simulink model "MC_R2_SFC_RELOJ_sin_antisway"  (R2025b)
settings: Solver=ode23t  StartTime=0.0  StopTime=600  MaxStep=T_s  RelTol=1e-4
InitFcn:
  | addpath(fileparts(get_param(bdroot,'FileName')),'-begin');
  | run(fullfile(fileparts(get_param(bdroot,'FileName')),'definir_buses_variadores.m'));
  | run(fullfile(fileparts(get_param(bdroot,'FileName')),'parametros_ganancias_cascada_29072026.m'));
  | run(fullfile(fileparts(get_param(bdroot,'FileName')),'configurar_modelo_final_hmi.m'));
  | run(fullfile(fileparts(get_param(bdroot,'FileName')),'configurar_parametros_variadores.m'));
  | Pvis.Ts_viz=0.04;Pvis.hmi.testDriver=@operador_medio_ciclo;
StopFcn:
  | cerrar_video_ensayo;
values from neighbouring files (symbols this model uses):
  MC_FF = struct('Ts',T_s,'gravity',g,'r_td',r_td,'i_t',i_t,'M_EQt',M_EQt,   'b_EQt',b_EQt,'Kx',K_x_cas,'Kp',K_pv_cas,'Ki',K_iv_cas,   'vmax',v_tmax,'amax',dv_tmax,'Imax',dv_tmax/K_iv_cas,   'r_hd',r_hd,'i_h',i_h,'M_EQh',M_EQh,'b_EQh',b_EQh,   'Khp',K_hp,'Khi',K_hi,'Khd',K_hd,'length0',l_hi,'swayOnTime',T_SW_on,   'swayFFRate',0.25,'observerWn',40.0,'observerZeta',1.0)    [configurar_parametros_variadores.m]
undefined symbols (not defined in the file or in its folder): b_cx, b_cy, b_hb, b_hEb, b_heq, b_t, b_tb, b_teq, b_tw, b_wu, g, H_c, HMI, i_h, i_t, J_heq, J_teq, K_cy, K_tw, k_wu, L_h0, l_hi, M_c_profile, M_s, M_t, nLevels0, omega_hmRATED, r_hd, r_td, slotBlock, T_hbMax, T_hEbMax, T_hmMax, T_s, T_s1, T_tbMax, T_tmMax, tau_hm, tau_tm, traj_duration, traj_x_start, traj_x_target, v_hmaxLoaded, v_hmaxUnloaded, x_tmax, x_tmin, Y_c0, Y_t0, Zbase
libraries: simulink x1, aerolibanimutils x1
(part 1 of 3)
Description:
  | Copia del modelo final con visualizacion y HMI integrada. Destino solo X, perfil LiDAR interno, offset de dos contenedores. Interfaz pasiva; retencion de barrido en supervisor. Correccion de ciclo: lazo de posicion de izaje, geometria real de slots, espera de alineacion/estabilidad y masa enclavada al PICK. Correccion de ciclo: lazo de posicion de izaje, geometria real de slots, espera de alineacion/estabilidad y masa enclavada al PICK. Correccion de ciclo: lazo de posicion de izaje, geometria real de slots, espera de alineacion/estabilidad y masa enclavada al PICK. Correccion de ciclo: lazo de posicion de izaje, geometria real de slots, espera de alineacion/estabilidad y masa enclavada al PICK. Correccion de ciclo: lazo de posicion de izaje, geometria real de slots, espera de alineacion/estabilidad y masa enclavada al PICK. Correccion de ciclo: lazo de posicion de izaje, geometria real de slots, espera de alineacion/estabilidad y masa enclavada al PICK. Correccion de ciclo: lazo de posicion de izaje, geometria real de slots, espera de alineacion/estabilidad y masa enclavada al PICK. Correccion de ciclo: lazo de posicion de izaje, geometria real de slots, espera de alineacion/estabilidad y masa enclavada al PICK. Correccion de ciclo: lazo de posicion de izaje, geometria real de slots, espera de alineacion/estabilidad y masa enclavada al PICK. Correccion de ciclo: lazo de posicion de izaje, geometria real de slots, espera de alineacion/estabilidad y masa enclavada al PICK. Correccion de ciclo: lazo de posicion de izaje, geometria real de slots, espera de alineacion/estabilidad y masa enclavada al PICK. Correccion de ciclo: lazo de posicion de izaje, geometria real de slots, espera de alineacion/estabilidad y masa enclavada al PICK.
  | Traslado productivo: 4 m/s y antisway inhibido durante transito con despeje confirmado.
  | Traslado productivo: 2.5 m/s y antisway inhibido durante crucero con despeje confirmado.
  | Traslado productivo: 2.5 m/s y antisway inhibido durante crucero con despeje confirmado.
settings Model: SimulationMode=accelerator  PacingRate=2  Creator=matie  LastModifiedBy=meesc
settings SolverCC: ZeroCrossAlgorithm=Adaptive  AlgebraicLoopSolver=TrustRegion
settings DataIOCC: SaveOutput=off  SaveTime=off
settings OptimizationCC: SimCompilerOptimization=on
settings DebuggingCC: IgnoredZcDiagnostic=none  UnconnectedInputMsg=warning  UnconnectedOutputMsg=warning  UnconnectedLineMsg=warning  BusObjectLabelMismatch=error
settings ModelReferenceCC: EnableRefExpFcnMdlSchedulingChecks=on
settings RTWCC: GPUComputeCapability=3.5
settings ConfigComp: PLC_OutputDir=C:\Temp\PLC_Code  PLC_TargetIDE=codesys23  PLC_MultiTBSigbuilderTimeRange=off  PLC_FoldFBCallOutputVar=off  PLC_RemoveUnusedSSMethodCallArguments=off  PLC_UseCallOutputArgSyntax=off  PLC_EnableUnsignedAndDoubleTypes=off  PLC_EnableUDTSplitting=off  PLC_MaxFieldsInUDT=500.0  PLC_InlineEnumCastFunction=off  PLC_RTWMaxIdLength=31.0  PLC_RollThreshold=5.0  PLC_ActiveTab=0.0  PLC_EnableStringLiteralTB=on  PLC_Enable64bitIntSupport=off

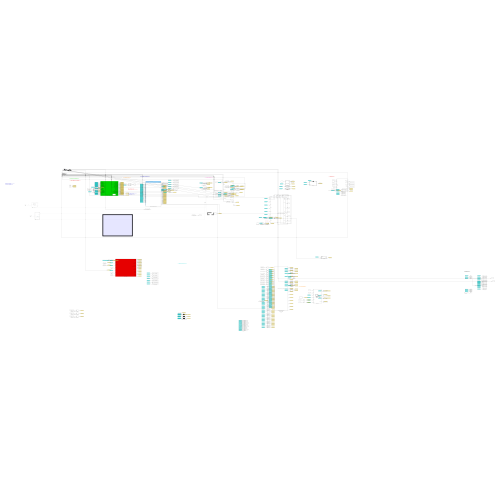
[thumbnail: Simulink's stored preview of the top-level diagram]
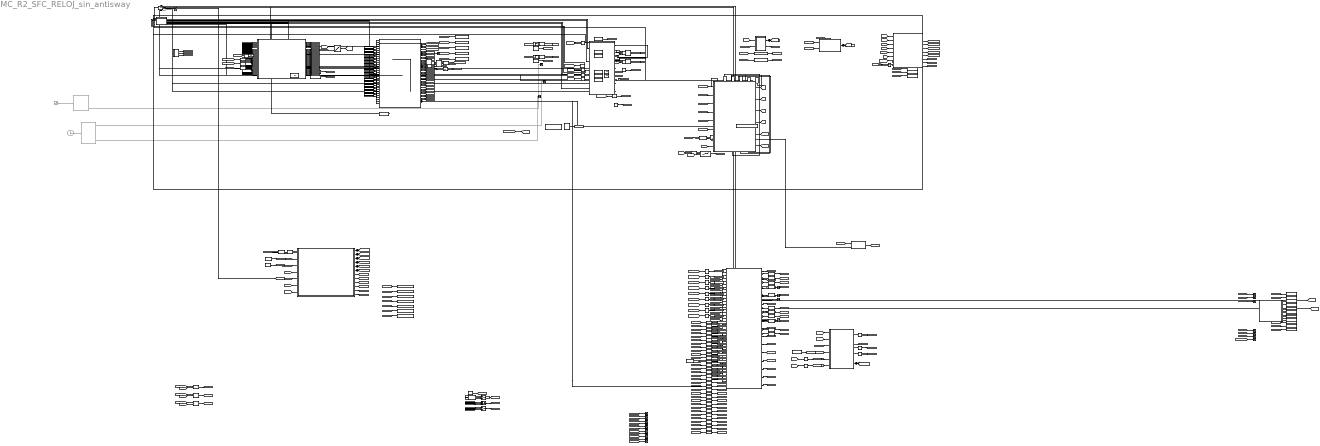
== system MC_R2_SFC_RELOJ_sin_antisway ==
  note: ESTIMADORES - OBSERVADORES
  note: INTEGRACION DEL SUPERVISOR
      | - Reemplaza exclusivamente Generador de trayectorias
      | - Conserva bloques comentados/no utilizados
      | - Ts supervisor: 20 ms; reguladores: 10 ms
  note: NIVEL 0 - SEGURIDAD (Ts = 20 ms)
      | E-stop/watchdog: emergencia total
      | Limite ultimo/sobrevelocidad: aislamiento selectivo por eje
  note: NIVEL 1 CORREGIDO - 2026-08-20
      | - Arranque automatico y planificador de obstaculos
      | - Transferencias bumpless
      | - Apertura de twistlocks y frenado seguro
  note: === INTERFAZ DE ENTRADAS ===
  note: === AUTOMATA SUPERVISOR ===
  note: === CONTROLADORES ===
  note: === PLANTA Y PERFIL ===
  note: === SENSORES ===
  note: === VISUALIZACION + HMI ===
  note: === AUTOMATA DE SEGURIDAD ===
  note: === TOMA / ENTREGA ===
  note: === MONITOREO ===
  1-D Lookup Table : Lookup_n-D  NumberOfTableDimensions=1  BreakpointsForDimension1=-30 + (0:32)*2.44  TableSource=Input port  Table=tanh([-5:5])  InterpMethod=Flat  InternalRulePriority=Speed  RndMeth=Simplest
      settings: InputPortMap=u0,p221
  Actualizar_Yc : Subsystem
  Altura cambio a automatico : Constant  Value=HMI.manualToAutoHeight
  Automata Supervisor : Subsystem
  Clock : Clock  Commented=on
  Consigna Izaje : MATLAB Function  Commented=on  TreatAsAtomicUnit=on
  Constant : Constant  Value=0
  Constant1 : Constant
  Constant2 : Constant  Value=l_hi
  Constant4 : Constant  Value=slotBlock
  Constant5 : Constant  Value=0
  Distancia aproximacion manual : Constant  Value=HMI.finalApproachDistance
  Estados MC carro : BusSelector  OutputSignals=x,omegaDrum,velocity,observerAngle
  Estados MC izaje : BusSelector  OutputSignals=length,lengthRate,omegaDrum,observerAngle
  HMI_COLISION_NO_DISPONIBLE : Constant  Value=NaN
  HMI_ESTADO_{10..41} (32 alike) : ZeroOrderHold  SampleTime=Pvis.Ts_viz
  HMI_MANDO_01 : DataTypeConversion  OutDataTypeStr=boolean  SaturateOnIntegerOverflow=off  RndMeth=Floor
  HMI_MANDO_02 : DataTypeConversion  OutDataTypeStr=boolean  SaturateOnIntegerOverflow=off  RndMeth=Floor
  HMI_MANDO_03 : DataTypeConversion  OutDataTypeStr=boolean  SaturateOnIntegerOverflow=off  RndMeth=Floor
  HMI_MANDO_04 : DataTypeConversion  OutDataTypeStr=boolean  SaturateOnIntegerOverflow=off  RndMeth=Floor
  HMI_MANDO_06 : DataTypeConversion  OutDataTypeStr=double  SaturateOnIntegerOverflow=off  RndMeth=Floor
  HMI_MANDO_09 : DataTypeConversion  OutDataTypeStr=boolean  SaturateOnIntegerOverflow=off  RndMeth=Floor
  HMI_MANDO_10 : DataTypeConversion  OutDataTypeStr=boolean  SaturateOnIntegerOverflow=off  RndMeth=Floor
  HMI_MANDO_11 : DataTypeConversion  OutDataTypeStr=boolean  SaturateOnIntegerOverflow=off  RndMeth=Floor
  HMI_MANDO_12 : DataTypeConversion  OutDataTypeStr=double  SaturateOnIntegerOverflow=off  RndMeth=Floor
  HMI_MANDO_14 : DataTypeConversion  OutDataTypeStr=double  SaturateOnIntegerOverflow=off  RndMeth=Floor
  HMI_MANDO_15 : DataTypeConversion  OutDataTypeStr=double  SaturateOnIntegerOverflow=off  RndMeth=Floor
  HMI_RESERVA_05 : Terminator
  HMI_RESERVA_07 : Terminator
  HMI_RESERVA_08 : Terminator
  HMI_RESERVA_13 : Terminator
  HMI_SELECT_JOY_H : Switch  Criteria=u2 > Threshold  Threshold=0.5  SaturateOnIntegerOverflow=off  InputSameDT=off
  HMI_SELECT_JOY_T : Switch  Criteria=u2 > Threshold  Threshold=0.5  SaturateOnIntegerOverflow=off  InputSameDT=off
  HMI_SELECT_TWIST_BUTTON : Switch  Criteria=u2 > Threshold  Threshold=0.5  SaturateOnIntegerOverflow=off  InputSameDT=off
  HMI_USE_JOYSTICK : Constant  Value=double(HMI.useJoystick)
  HMI_ZERO_INPUT : Constant  Value=0.0
  Habilitacion par izaje : Product  Inputs=**
  Habilitacion par trolley : Product  Inputs=**
  Histeresis_F_hw : MATLAB Function  TreatAsAtomicUnit=on
  Histeresis_contacto : MATLAB Function  TreatAsAtomicUnit=on
  Interfaz MC : Subsystem
  Interfaz de entradas del supervisor : Subsystem  Description=Interfaz pasiva: 33 conexiones directas Inport-Outport. Todo calculo y enclavamiento pertenece al automata supervisor.
  LIDAR_OFFSET_X : Bias  Bias=HMI.lidarOffsetX  SaturateOnIntegerOverflow=off
  LIDAR_PROFILE_LOOKUP : Lookup_n-D  NumberOfTableDimensions=1  BreakpointsForDimension1=-30 + (0:32)*2.44  TableSource=Input port  Table=tanh([-5:5])  InterpMethod=Flat  InternalRulePriority=Speed  RndMeth=Simplest
      settings: InputPortMap=u0,p221
  LOG_mon_aHoistMeasured : ToWorkspace  VariableName=mon_aHoistMeasured  SaveFormat=Timeseries  SampleTime=-1
  LOG_mon_aTrolleyMeasured : ToWorkspace  VariableName=mon_aTrolleyMeasured  SaveFormat=Timeseries  SampleTime=-1
  LOG_mon_automaticTargetY : ToWorkspace  VariableName=mon_automaticTargetY  SaveFormat=Timeseries  SampleTime=-1
  LOG_mon_ayRef : ToWorkspace  VariableName=mon_ayRef  SaveFormat=Timeseries  SampleTime=-1
  LOG_mon_contact4 : ToWorkspace  VariableName=mon_contact4  SaveFormat=Timeseries  SampleTime=-1
  LOG_mon_lidarX : ToWorkspace  VariableName=mon_lidarX  SaveFormat=Timeseries  SampleTime=-1
  LOG_mon_lidarY : ToWorkspace  VariableName=mon_lidarY  SaveFormat=Timeseries  SampleTime=-1
  LOG_mon_profileMaxY : ToWorkspace  VariableName=mon_profileMaxY  SaveFormat=Timeseries  SampleTime=-1
  LOG_mon_profileScanComplete : ToWorkspace  VariableName=mon_profileScanComplete  SaveFormat=Timeseries  SampleTime=-1
  LOG_mon_profileValid : ToWorkspace  VariableName=mon_profileValid  SaveFormat=Timeseries  SampleTime=-1
  LOG_mon_scanActive : ToWorkspace  VariableName=mon_scanActive  SaveFormat=Timeseries  SampleTime=-1
  LOG_mon_scannedObstacleProfile : ToWorkspace  VariableName=mon_scannedObstacleProfile  SaveFormat=Timeseries  SampleTime=-1
  LOG_mon_swayEnable : ToWorkspace  VariableName=mon_swayEnable  SaveFormat=Timeseries  SampleTime=-1
  LOG_mon_torqueProvenHoist : ToWorkspace  VariableName=mon_torqueProvenHoist  SaveFormat=Timeseries  SampleTime=-1
  LOG_mon_torqueProvenTrolley : ToWorkspace  VariableName=mon_torqueProvenTrolley  SaveFormat=Timeseries  SampleTime=-1
  LOG_mon_trackingFault : ToWorkspace  VariableName=mon_trackingFault  SaveFormat=Timeseries  SampleTime=-1
  LOG_mon_twistlockCloseCmd : ToWorkspace  VariableName=mon_twistlockCloseCmd  SaveFormat=Timeseries  SampleTime=-1
  LOG_mon_twistlocksClosed : ToWorkspace  VariableName=mon_twistlocksClosed  SaveFormat=Timeseries  SampleTime=-1
  LOG_mon_vyRef : ToWorkspace  VariableName=mon_vyRef  SaveFormat=Timeseries  SampleTime=-1
  LOG_mon_yRef : ToWorkspace  VariableName=mon_yRef  SaveFormat=Timeseries  SampleTime=-1
  LOG_n0_brakeHoistOpen : ToWorkspace  VariableName=n0_brakeHoistOpen  SaveFormat=Timeseries  SampleTime=-1
  LOG_n0_brakeTrolleyOpen : ToWorkspace  VariableName=n0_brakeTrolleyOpen  SaveFormat=Timeseries  SampleTime=-1
  LOG_n0_emergency : ToWorkspace  VariableName=n0_emergency  SaveFormat=Timeseries  SampleTime=-1
  LOG_n0_emergencyBrakeHoistOpen : ToWorkspace  VariableName=n0_emergencyBrakeHoistOpen  SaveFormat=Timeseries  SampleTime=-1
  LOG_n0_permitGlobal : ToWorkspace  VariableName=n0_permitGlobal  SaveFormat=Timeseries  SampleTime=-1
  LOG_n0_permitHoist : ToWorkspace  VariableName=n0_permitHoist  SaveFormat=Timeseries  SampleTime=-1
  LOG_n0_permitTrolley : ToWorkspace  VariableName=n0_permitTrolley  SaveFormat=Timeseries  SampleTime=-1
  LOG_sup_alarmCode : ToWorkspace  VariableName=sup_alarmCode  SaveFormat=Timeseries  SampleTime=-1
  LOG_sup_faultCode : ToWorkspace  VariableName=sup_faultCode  SaveFormat=Timeseries  SampleTime=-1
  LOG_sup_loadedState : ToWorkspace  VariableName=sup_loadedState  SaveFormat=Timeseries  SampleTime=-1
  LOG_sup_modeCode : ToWorkspace  VariableName=sup_modeCode  SaveFormat=Timeseries  SampleTime=-1
  LOG_sup_overloadDetected : ToWorkspace  VariableName=sup_overloadDetected  SaveFormat=Timeseries  SampleTime=-1
  MASS_latch_pick : MATLAB Function  TreatAsAtomicUnit=on
  MASS_loaded_gate : Product  Inputs=**
  MASS_profile_lookup : Lookup_n-D  NumberOfTableDimensions=1  BreakpointsForDimension1=1:33  Table=M_c_profile  InterpMethod=Flat  ExtrapMethod=Clip  InternalRulePriority=Speed  RndMeth=Simplest
  MASS_slot_double : DataTypeConversion  OutDataTypeStr=double  SaturateOnIntegerOverflow=off  RndMeth=Floor
  MONITOR_REQUISITOS : Subsystem
  Memoria recorte torque AW : UnitDelay  SampleTime=T_s  HasFrameUpgradeWarning=on
  Memory : Memory  InheritSampleTime=on
  Memory1 : Memory  InheritSampleTime=on
  Memory2 : Memory  InheritSampleTime=on
  Monitor bus diagnosticos 6 : Terminator
  Monitor bus diagnosticos 7 : Terminator
  Monitor estado carro {1..4} (4 alike) : Terminator
  Monitor estado izaje {1..4} (4 alike) : Terminator
  Motion Controller : Subsystem
  N0_CMD_ESTOP : Constant  Value=false  OutDataTypeStr=boolean
  N0_CMD_RESET : Constant  Value=false  OutDataTypeStr=boolean
  N0_GATE_BRK_H : Logic  AllPortsSameDT=off  OutDataTypeStr=boolean
  N0_GATE_BRK_HE : Logic  AllPortsSameDT=off  OutDataTypeStr=boolean
  N0_GATE_BRK_T : Logic  AllPortsSameDT=off  OutDataTypeStr=boolean
  N0_WATCHDOG_DELAY : UnitDelay  SampleTime=0.02  HasFrameUpgradeWarning=on
  N0_WATCHDOG_DOUBLE : DataTypeConversion  OutDataTypeStr=boolean  SaturateOnIntegerOverflow=off  RndMeth=Floor
  Nivel 0 - Seguridad : Subsystem
  PICK / PLACE : Stateflow chart  TreatAsAtomicUnit=on
      settings: PortSchema="{\"entries\":[{\"content\":{\"sides\":[{\"content\":{\"connectorIds\":[\"In1\",\"In4\",\"In2\",\"In3\",\"In5\",\"In6\"]},\"type\":\"ConnectorPlacement.EquallySpacedRectSide\",\"uuid\":\"a5c16d2a-5865-4365-aaee-c28e35544d9c\"},{\"content\":{\"connectorIds\":[\"Out1\",\"Out2\",\"Out3\",\"Out4\"],\"side\":\"RIGHT\"},\"type\":\"ConnectorPlacement.EquallySpacedRectSide\",\"uuid\":\"08faef91-0dc9-4101-b812-f759fd3bf652\"},{\"content\":{\"side\":\"TOP\"},\"type\":\"ConnectorPlacement.EquallySpacedRectSide\",\"uuid\":\"3d592ef8-c17c-453f-9fe4-450a9042f638\"}]},\"type\":\"ConnectorPlacement.EquallySpacedConnector\",\"uuid\":\"5bde2fb2-ef6e-4078-a945-4a946a0492f9\"}],\"packageUris\":[\"http://schema.mathworks.com/mf0/Connector/R2020b\"],\"version\":\"1.0\"}"
  Planta : Subsystem
      settings: PortSchema="{\"entries\":[{\"content\":{\"sides\":[{\"content\":{\"connectorIds\":[\"In1\",\"In2\",\"In3\",\"In4\",\"In5\",\"In6\",\"In7\",\"In8\"]},\"type\":\"ConnectorPlacement.EquallySpacedRectSide\",\"uuid\":\"5d76959f-b6a9-444d-8994-ab0bade83e0d\"},{\"content\":{\"connectorIds\":[\"Out1\",\"Out2\",\"Out3\",\"Out4\",\"Out5\",\"Out6\"],\"side\":\"RIGHT\"},\"type\":\"ConnectorPlacement.EquallySpacedRectSide\",\"uuid\":\"6304bef6-506d-485c-ab14-4271018549da\"},{\"content\":{\"connectorIds\":[\"Out7\",\"Out8\",\"Out9\",\"Out10\",\"Out11\",\"Out12\"],\"side\":\"TOP\"},\"type\":\"ConnectorPlacement.EquallySpacedRectSide\",\"uuid\":\"df87386f-05e1-445d-949d-2fc2ff55887c\"},{\"content\":{\"side\":\"BOTTOM\"},\"type\":\"ConnectorPlacement.EquallySpacedRectSide\",\"uuid\":\"6e66bc8d-e30f-453c-8c56-304efc1d1a44\"}]},\"type\":\"ConnectorPlacement.EquallySpacedConnector\",\"uuid\":\"ae511e70-0859-4f7f-ad0a-8f37dd26c1e0\"}],\"packageUris\":[\"http://schema.mathworks.com/mf0/Connector/R2020b\"],\"version\":\"1.0\"}"
  Push Button : PushButtonBlock  ButtonType=Latch  IconOnColor=[0.0, 0.39215686274509803, 0.0]  IconOffColor=[0.0, 1.0, 0.0]  OffValue=0.000000
  Registrar_envolvente_seguridad : ToWorkspace  VariableName=mon_safetyEnvelopeProfile  SaveFormat=Timeseries  SampleTime=-1
  SENSORES : Subsystem
  SUP_AUTO_TARGET_X_RAW : Constant  Value=HMI.shipTargetX  OutDataTypeStr=double
  SUP_CMD_AUTO_START_RAW : DataTypeConversion  OutDataTypeStr=boolean  SaturateOnIntegerOverflow=off  RndMeth=Floor
  SUP_CMD_AUTO_START_RAW_STEP : Step  Time=0.5  SampleTime=0
  SUP_CMD_RESET_RAW : Constant  Value=false  OutDataTypeStr=boolean
  SUP_CMD_START_RAW : DataTypeConversion  OutDataTypeStr=boolean  SaturateOnIntegerOverflow=off  RndMeth=Floor
  SUP_CMD_START_RAW_STEP : Step  Time=0.1  SampleTime=0
  SUP_CMD_STOP_RAW : Constant  Value=false  OutDataTypeStr=boolean
  SUP_CONFIG_VALID_RAW : Constant  Value=HMI.configValid  OutDataTypeStr=boolean
  SUP_CONTACT_BOOL : DataTypeConversion  OutDataTypeStr=boolean  SaturateOnIntegerOverflow=off  RndMeth=Floor
  SUP_FB_BOOL_7 : DataTypeConversion  OutDataTypeStr=boolean  SaturateOnIntegerOverflow=off  RndMeth=Floor
  SUP_FB_BOOL_8 : DataTypeConversion  OutDataTypeStr=boolean  SaturateOnIntegerOverflow=off  RndMeth=Floor
  SUP_MODE_AUTO_REQ_RAW : Constant  Value=HMI.modeAutoReq  OutDataTypeStr=boolean
  SUP_NOT_OPEN : Logic  Operator=NOT  AllPortsSameDT=off  OutDataTypeStr=boolean
  SUP_SCAN_PROFILE_REQ_RAW : Constant  Value=HMI.scanProfileReq  OutDataTypeStr=boolean
  SUP_SCAN_SPEED_RAW : Constant  Value=HMI.scanSpeed  OutDataTypeStr=double
  SUP_SWAY_SELECT_RAW : Constant  Value=HMI.swayControlSelect  OutDataTypeStr=boolean
  SUP_TLK_DOUBLE : DataTypeConversion  OutDataTypeStr=double  SaturateOnIntegerOverflow=off  RndMeth=Floor
  SUP_TLK_MEMORIA : UnitDelay  SampleTime=0.02  HasFrameUpgradeWarning=on
  SUP_TLK_SET_OR : Logic  Operator=OR  AllPortsSameDT=off  OutDataTypeStr=boolean
  SUP_TORQUE_HOIST_Z1 : UnitDelay  SampleTime=T_s1  HasFrameUpgradeWarning=on
  SUP_TORQUE_TROLLEY_Z1 : UnitDelay  SampleTime=T_s1  HasFrameUpgradeWarning=on
  SUP_TWISTLOCK_CMD : Logic  AllPortsSameDT=off  OutDataTypeStr=boolean
  SUP_TWISTLOCK_FB_DELAY : UnitDelay  SampleTime=0.02  HasFrameUpgradeWarning=on
  SW ultima muestra N1 : UnitDelay  SampleTime=T_s1  HasFrameUpgradeWarning=on
  Step : Step  Commented=on  Time=4  SampleTime=0
  Subsystem1 : Subsystem
  TERM_Constant : Terminator
  TERM_Constant1 : Terminator
  TERM_Constant5 : Terminator
  TERM_HMI_HMI_SELECT_JOY_H : Terminator
  TERM_HMI_HMI_SELECT_JOY_T : Terminator
  TERM_HMI_HMI_SELECT_TWIST_BUTTON : Terminator
  TERM_HMI_N0_CMD_ESTOP : Terminator
  TERM_HMI_N0_CMD_RESET : Terminator
  TERM_HMI_SUP_AUTO_TARGET_X_RAW : Terminator
  TERM_HMI_SUP_CMD_AUTO_START_RAW : Terminator
  TERM_HMI_SUP_CMD_RESET_RAW : Terminator
  TERM_HMI_SUP_CMD_START_RAW : Terminator
  TERM_HMI_SUP_CMD_STOP_RAW : Terminator
  TERM_HMI_SUP_MODE_AUTO_REQ_RAW : Terminator
  TERM_HMI_SUP_SCAN_PROFILE_REQ_RAW : Terminator
  TERM_SENSOR_08 : Terminator
  TERM_SENSOR_09 : Terminator
  TERM_SENSOR_10 : Terminator
  TERM_SUP_FB_6 : Terminator
  Terminator{2..5} (4 alike) : Terminator
  Transferencia antisway no transmitida : Terminator
  Transferencia no implementada PLC anterior : Constant  Value=0
  Trayectoria : Stateflow chart  Commented=on  TreatAsAtomicUnit=on  SystemSampleTime=1e-2
      settings: PortSchema="{\"entries\":[{\"content\":{\"sides\":[{\"content\":{\"connectorIds\":[\"In1\"]},\"type\":\"ConnectorPlacement.EquallySpacedRectSide\",\"uuid\":\"6f391abb-7914-46b1-bf75-00dd597d8745\"},{\"content\":{\"connectorIds\":[\"Out2\",\"Out1\",\"Out3\",\"Out4\"],\"side\":\"RIGHT\"},\"type\":\"ConnectorPlacement.EquallySpacedRectSide\",\"uuid\":\"48dcce50-4b02-4ca8-9f00-9379aa6a7819\"},{\"content\":{\"side\":\"TOP\"},\"type\":\"ConnectorPlacement.EquallySpacedRectSide\",\"uuid\":\"d392ffd4-6ceb-4d84-99b2-b6bd8ae66add\"}]},\"type\":\"ConnectorPlacement.EquallySpacedConnector\",\"uuid\":\"17183b69-1a6f-4f40-a08d-c34759601e28\"}],\"packageUris\":[\"http://schema.mathworks.com/mf0/Connector/R2020b\"],\"version\":\"1.0\"}"
  Unit Delay : UnitDelay  SampleTime=-1  HasFrameUpgradeWarning=on
  Unit Delay1 : UnitDelay  SampleTime=-1  HasFrameUpgradeWarning=on
  VIS ZOH 01 : ZeroOrderHold  SampleTime=Pvis.Ts_viz
  VIS ZOH 02 : ZeroOrderHold  SampleTime=Pvis.Ts_viz
  VIS ZOH 03 : ZeroOrderHold  SampleTime=Pvis.Ts_viz
  VIS ZOH 04 : ZeroOrderHold  SampleTime=Pvis.Ts_viz
  VIS ZOH 05 : ZeroOrderHold  SampleTime=Pvis.Ts_viz
  VIS ZOH 06 : ZeroOrderHold  SampleTime=Pvis.Ts_viz
  VIS ZOH 07 : ZeroOrderHold  SampleTime=Pvis.Ts_viz
  VIS ZOH 08 : ZeroOrderHold  SampleTime=Pvis.Ts_viz
  VIS ZOH 09 : ZeroOrderHold  SampleTime=Pvis.Ts_viz
  VISUALIZACION 2D SISTEMA GRUA : M-S-Function  FunctionName=visualizacion_modelo_final_hmi_corregido
      settings: AttributesFormatString=Grua + HMI interactiva\n41 estados / 15 mandos\nTs = 40 ms
  Zero-Order Hold{,5..10} (7 alike) : ZeroOrderHold  SampleTime=T_s
  Zero-Order Hold11 : ZeroOrderHold  SampleTime=0.001
  Zero-Order Hold12 : ZeroOrderHold  SampleTime=0.001
  slot_x_l : MATLAB Function  TreatAsAtomicUnit=on
  tag scope: F_hw=global, N0_BRK_H=global, N0_BRK_HE=global, N0_BRK_T=global, N0_PERMIT_GLOBAL=global, N0_PERMIT_HOIST=global, N0_PERMIT_TROLLEY=global, Y_c=global, a_tgen=global, carga_tomada=global, k_slot=global, omega_l=global, theta_l=global, v_ly=global, v_tgen=global, x_t=global, x_tgen=global, y_l=global
  wires:
  Step/1 -> Trayectoria/1(iniciar)  "start"
  Trayectoria/4(j_act) -> Terminator5/1
  1-D Lookup Table/1 -> [yc_xl]
  Clock/1 -> Consigna Izaje/1(t)
  Consigna Izaje/1(lh_ref) -> Terminator2/1  "lh_ref"
  Consigna Izaje/4(done) -> Terminator4/1
  Actualizar_Yc/1(Y_c) -> [Y_c], [TOP_Actualizar_Yc_P1]
  Altura cambio a automatico/1 -> [TOP_Altura_cambio_a_automatico_P1]
  Constant/1 -> [TOP_Constant_P1]
  Constant1/1 -> [TOP_Constant1_P1]
  Constant4/1 -> [TOP_Constant4_P1]
  Constant5/1 -> [TOP_Constant5_P1]
  Distancia aproximacion manual/1 -> [TOP_Distancia_aproximacion_manual_P1]
  [theta_l_sens] -> Zero-Order Hold5/1
  [F_hw] -> Zero-Order Hold12/1
  [yc_xl] -> Planta/8(y_c0(x_l,t))  "yc_xl"
  [x_l] -> slot_x_l/1(x_l)
  [x_l] -> 1-D Lookup Table/1
  [x_tgen] -> Zero-Order Hold6/1
  [carga_tomada] -> Unit Delay/1
  [TLK] -> PICK / PLACE/1(TLK)
  [theta_l] -> SENSORES/4(theta_l)
  [x_t] -> SENSORES/6(x_t)
  [omega_hd] -> SENSORES/7(In7)
  [theta_tm] -> SENSORES/1(In1)
  [theta_hm] -> SENSORES/2(In2)
  [F_hw] -> SENSORES/3(In3)
  [v_tgen] -> Zero-Order Hold7/1
  [omega_l] -> SENSORES/5(omega_l)
  [carga_tomada] -> Unit Delay1/1
  [v_ly] -> PICK / PLACE/4(v_yl)
  [F_cy] -> Zero-Order Hold11/1
  [a_tgen] -> Zero-Order Hold8/1
  [F_hw_sens] -> Zero-Order Hold/1
  [TOP_Actualizar_Yc_P1] -> 1-D Lookup Table/2
  [TOP_Altura_cambio_a_automatico_P1] -> Interfaz de entradas del supervisor/26(IN_26_manualToAutoHeight)
  [TOP_Automata_Supervisor_P10] -> HMI_ESTADO_23/1
  [TOP_Automata_Supervisor_P10] -> LOG_sup_overloadDetected/1
  [TOP_Automata_Supervisor_P11] -> N0_WATCHDOG_DOUBLE/1
  [TOP_Automata_Supervisor_P15] -> LOG_mon_yRef/1
  [TOP_Automata_Supervisor_P15] -> Terminator3/1
  [TOP_Automata_Supervisor_P16] -> LOG_mon_vyRef/1
  [TOP_Automata_Supervisor_P17] -> LOG_mon_ayRef/1
  [TOP_Automata_Supervisor_P18] -> HMI_ESTADO_10/1
  [TOP_Automata_Supervisor_P18] -> LOG_sup_modeCode/1
  [TOP_Automata_Supervisor_P19] -> LOG_sup_alarmCode/1
  [TOP_Automata_Supervisor_P20] -> HMI_ESTADO_40/1
  [TOP_Automata_Supervisor_P20] -> LOG_sup_faultCode/1
  [TOP_Automata_Supervisor_P21] -> LOG_mon_aTrolleyMeasured/1
  [TOP_Automata_Supervisor_P22] -> LOG_mon_aHoistMeasured/1
  [TOP_Automata_Supervisor_P23] -> HMI_ESTADO_39/1
  [TOP_Automata_Supervisor_P23] -> LOG_mon_trackingFault/1
  [TOP_Automata_Supervisor_P24] -> LOG_mon_torqueProvenTrolley/1
  [TOP_Automata_Supervisor_P25] -> LOG_mon_torqueProvenHoist/1
  [TOP_Automata_Supervisor_P26] -> HMI_ESTADO_41/1
  [TOP_Automata_Supervisor_P26] -> LOG_mon_profileScanComplete/1
  [TOP_Automata_Supervisor_P27] -> HMI_ESTADO_37/1
  [TOP_Automata_Supervisor_P27] -> LOG_mon_profileValid/1
  [TOP_Automata_Supervisor_P28] -> HMI_ESTADO_38/1
  [TOP_Automata_Supervisor_P28] -> LOG_mon_scanActive/1
  [TOP_Automata_Supervisor_P29] -> LOG_mon_scannedObstacleProfile/1
  [TOP_Automata_Supervisor_P30] -> LOG_mon_profileMaxY/1
  [TOP_Automata_Supervisor_P31] -> HMI_ESTADO_36/1
  [TOP_Automata_Supervisor_P31] -> LOG_mon_automaticTargetY/1
  [TOP_Automata_Supervisor_P32] -> HMI_ESTADO_35/1
  [TOP_Automata_Supervisor_P33] -> HMI_ESTADO_12/1
  [TOP_Automata_Supervisor_P34] -> HMI_ESTADO_13/1
  [TOP_Automata_Supervisor_P35] -> HMI_ESTADO_26/1
  [TOP_Automata_Supervisor_P36] -> HMI_ESTADO_27/1
  [TOP_Automata_Supervisor_P37] -> HMI_ESTADO_20/1
  [TOP_Automata_Supervisor_P38] -> HMI_ESTADO_21/1
  [TOP_Automata_Supervisor_P6] -> LOG_mon_twistlockCloseCmd/1
  [TOP_Automata_Supervisor_P6] -> SUP_TLK_SET_OR/1
  [TOP_Automata_Supervisor_P7] -> SUP_NOT_OPEN/1
  [TOP_Automata_Supervisor_P8] -> HMI_ESTADO_14/1
  [TOP_Automata_Supervisor_P8] -> LOG_mon_swayEnable/1
  [TOP_Automata_Supervisor_P9] -> LOG_sup_loadedState/1
  [TOP_Constant1_P1] -> TERM_Constant1/1
  [TOP_Constant4_P1] -> slot_x_l/2(slotBlock)
  [TOP_Constant5_P1] -> TERM_Constant5/1
  [TOP_Constant_P1] -> TERM_Constant/1
  [TOP_Distancia_aproximacion_manual_P1] -> Interfaz de entradas del supervisor/27(IN_27_finalApproachDistance)
  [TOP_HMI_COLISION_NO_DISPONIBLE_P1] -> HMI_ESTADO_28/1
  [TOP_HMI_ESTADO_10_P1] -> VISUALIZACION 2D SISTEMA GRUA/10
  [TOP_HMI_ESTADO_11_P1] -> VISUALIZACION 2D SISTEMA GRUA/11
  [TOP_HMI_ESTADO_12_P1] -> VISUALIZACION 2D SISTEMA GRUA/12
  [TOP_HMI_ESTADO_13_P1] -> VISUALIZACION 2D SISTEMA GRUA/13
  [TOP_HMI_ESTADO_14_P1] -> VISUALIZACION 2D SISTEMA GRUA/14
  [TOP_HMI_ESTADO_15_P1] -> VISUALIZACION 2D SISTEMA GRUA/15
  [TOP_HMI_ESTADO_16_P1] -> VISUALIZACION 2D SISTEMA GRUA/16
  [TOP_HMI_ESTADO_17_P1] -> VISUALIZACION 2D SISTEMA GRUA/17
  [TOP_HMI_ESTADO_18_P1] -> VISUALIZACION 2D SISTEMA GRUA/18
  [TOP_HMI_ESTADO_19_P1] -> VISUALIZACION 2D SISTEMA GRUA/19
  [TOP_HMI_ESTADO_20_P1] -> VISUALIZACION 2D SISTEMA GRUA/20
  [TOP_HMI_ESTADO_21_P1] -> VISUALIZACION 2D SISTEMA GRUA/21
  [TOP_HMI_ESTADO_22_P1] -> VISUALIZACION 2D SISTEMA GRUA/22
  [TOP_HMI_ESTADO_23_P1] -> VISUALIZACION 2D SISTEMA GRUA/23
  [TOP_HMI_ESTADO_24_P1] -> VISUALIZACION 2D SISTEMA GRUA/24
  [TOP_HMI_ESTADO_25_P1] -> VISUALIZACION 2D SISTEMA GRUA/25
  [TOP_HMI_ESTADO_26_P1] -> VISUALIZACION 2D SISTEMA GRUA/26
  [TOP_HMI_ESTADO_27_P1] -> VISUALIZACION 2D SISTEMA GRUA/27
  [TOP_HMI_ESTADO_28_P1] -> VISUALIZACION 2D SISTEMA GRUA/28
  [TOP_HMI_ESTADO_29_P1] -> VISUALIZACION 2D SISTEMA GRUA/29
  [TOP_HMI_ESTADO_30_P1] -> VISUALIZACION 2D SISTEMA GRUA/30
  [TOP_HMI_ESTADO_31_P1] -> VISUALIZACION 2D SISTEMA GRUA/31
  [TOP_HMI_ESTADO_32_P1] -> VISUALIZACION 2D SISTEMA GRUA/32
  [TOP_HMI_ESTADO_33_P1] -> VISUALIZACION 2D SISTEMA GRUA/33
  [TOP_HMI_ESTADO_34_P1] -> VISUALIZACION 2D SISTEMA GRUA/34
  [TOP_HMI_ESTADO_35_P1] -> VISUALIZACION 2D SISTEMA GRUA/35
  [TOP_HMI_ESTADO_36_P1] -> VISUALIZACION 2D SISTEMA GRUA/36
  [TOP_HMI_ESTADO_37_P1] -> VISUALIZACION 2D SISTEMA GRUA/37
  [TOP_HMI_ESTADO_38_P1] -> VISUALIZACION 2D SISTEMA GRUA/38
  [TOP_HMI_ESTADO_39_P1] -> VISUALIZACION 2D SISTEMA GRUA/39
  [TOP_HMI_ESTADO_40_P1] -> VISUALIZACION 2D SISTEMA GRUA/40
  [TOP_HMI_ESTADO_41_P1] -> VISUALIZACION 2D SISTEMA GRUA/41
  [TOP_HMI_MANDO_01_P1] -> Interfaz de entradas del supervisor/1(IN_01_cmdStart)
  [TOP_HMI_MANDO_02_P1] -> Interfaz de entradas del supervisor/2(IN_02_cmdStop)
  [TOP_HMI_MANDO_03_P1] -> Nivel 0 - Seguridad/3(emergencyStop)
  [TOP_HMI_MANDO_04_P1] -> Interfaz de entradas del supervisor/30(IN_30_scanProfileReq)
  [TOP_HMI_MANDO_06_P1] -> Interfaz de entradas del supervisor/25(IN_25_autoTargetX)
  [TOP_HMI_MANDO_09_P1] -> Interfaz de entradas del supervisor/3(IN_03_modeAutoReq)
  [TOP_HMI_MANDO_10_P1] -> Interfaz de entradas del supervisor/4(IN_04_cmdAutoStart)
  [TOP_HMI_MANDO_11_P1] -> Interfaz de entradas del supervisor/5(IN_05_cmdReset)
  [TOP_HMI_MANDO_11_P1] -> Nivel 0 - Seguridad/2(resetSafety)
  [TOP_HMI_MANDO_12_P1] -> Interfaz de entradas del supervisor/8(IN_08_twistlockButton)
  [TOP_HMI_MANDO_14_P1] -> Interfaz de entradas del supervisor/16(IN_16_joyTrolley)
  [TOP_HMI_MANDO_15_P1] -> Interfaz de entradas del supervisor/17(IN_17_joyHoist)
  [TOP_HMI_SELECT_JOY_H_P1] -> TERM_HMI_HMI_SELECT_JOY_H/1
  [TOP_HMI_SELECT_JOY_T_P1] -> TERM_HMI_HMI_SELECT_JOY_T/1
  [TOP_HMI_SELECT_TWIST_BUTTON_P1] -> TERM_HMI_HMI_SELECT_TWIST_BUTTON/1
  [TOP_HMI_USE_JOYSTICK_P1] -> HMI_SELECT_JOY_H/2
  [TOP_HMI_USE_JOYSTICK_P1] -> HMI_SELECT_JOY_T/2
  [TOP_HMI_USE_JOYSTICK_P1] -> HMI_SELECT_TWIST_BUTTON/2
  [TOP_HMI_ZERO_INPUT_P1] -> HMI_SELECT_JOY_H/3
  [TOP_HMI_ZERO_INPUT_P1] -> HMI_SELECT_JOY_T/3
  [TOP_HMI_ZERO_INPUT_P1] -> HMI_SELECT_TWIST_BUTTON/3
  [TOP_Habilitacion_par_izaje_P1] -> Planta/1(T_hm*)
  [TOP_Habilitacion_par_trolley_P1] -> Planta/2(T_tm*)
  [TOP_Histeresis_F_hw_P1] -> PICK / PLACE/6(tension)
  [TOP_Histeresis_contacto_P1] -> PICK / PLACE/5(contacto)
  [TOP_Histeresis_contacto_P1] -> SUP_CONTACT_BOOL/1
  [TOP_Interfaz_de_entradas_del_supervisor_P9] -> LOG_mon_contact4/1
  [TOP_Interfaz_de_entradas_del_supervisor_P9] -> HMI_ESTADO_11/1
  [TOP_Interfaz_de_entradas_del_supervisor_P10] -> LOG_mon_twistlocksClosed/1
  [TOP_Interfaz_de_entradas_del_supervisor_P11] -> HMI_ESTADO_24/1
  [TOP_Interfaz_de_entradas_del_supervisor_P12] -> HMI_ESTADO_25/1
  [TOP_Interfaz_de_entradas_del_supervisor_P16] -> HMI_ESTADO_18/1
  [TOP_Interfaz_de_entradas_del_supervisor_P17] -> HMI_ESTADO_19/1
  [TOP_Interfaz_de_entradas_del_supervisor_P3] -> HMI_ESTADO_30/1
  [TOP_Interfaz_de_entradas_del_supervisor_P31] -> LOG_mon_lidarX/1
  [TOP_Interfaz_de_entradas_del_supervisor_P32] -> LOG_mon_lidarY/1
  [TOP_LIDAR_OFFSET_X_P1] -> Interfaz de entradas del supervisor/31(IN_31_lidarX)
  [TOP_LIDAR_OFFSET_X_P1] -> LIDAR_PROFILE_LOOKUP/1
  [TOP_LIDAR_PROFILE_LOOKUP_P1] -> Interfaz de entradas del supervisor/32(IN_32_lidarY)
  [TOP_MASS_latch_pick_P1] -> MASS_loaded_gate/1
  [TOP_MASS_loaded_gate_P1] -> Planta/7(M_c)
  [TOP_MASS_profile_lookup_P1] -> MASS_latch_pick/1(profileMass)
  [TOP_MASS_slot_double_P1] -> MASS_profile_lookup/1
  [TOP_Memory1_P1] -> Actualizar_Yc/1(tipo_evento)
  [TOP_Memory2_P1] -> Actualizar_Yc/2(slot_evento)
  [TOP_Memory_P1] -> Actualizar_Yc/Trigger
  [TOP_N0_CMD_ESTOP_P1] -> TERM_HMI_N0_CMD_ESTOP/1
  [TOP_N0_CMD_RESET_P1] -> TERM_HMI_N0_CMD_RESET/1
  [TOP_N0_GATE_BRK_HE_P1] -> Planta/4(BRK_hE)
  [TOP_N0_GATE_BRK_H_P1] -> Planta/5(BRK_h)
  [TOP_N0_GATE_BRK_T_P1] -> Planta/3(BRK_t)
  [TOP_N0_OMEGA_A_VT_P1] -> Nivel 0 - Seguridad/5(vTrolley)
  [TOP_N0_WATCHDOG_DELAY_P1] -> Nivel 0 - Seguridad/1(watchdogPulse)
  [TOP_N0_WATCHDOG_DOUBLE_P1] -> N0_WATCHDOG_DELAY/1
  [TOP_Nivel_0_Seguridad_P10] -> HMI_ESTADO_32/1
  [TOP_Nivel_0_Seguridad_P11] -> HMI_ESTADO_33/1
  [TOP_Nivel_0_Seguridad_P12] -> HMI_ESTADO_34/1
  [TOP_Nivel_0_Seguridad_P1] -> LOG_n0_permitGlobal/1
  [TOP_Nivel_0_Seguridad_P2] -> LOG_n0_permitTrolley/1
  [TOP_Nivel_0_Seguridad_P3] -> LOG_n0_permitHoist/1
  [TOP_Nivel_0_Seguridad_P4] -> HMI_ESTADO_15/1
  [TOP_Nivel_0_Seguridad_P4] -> LOG_n0_brakeTrolleyOpen/1
  [TOP_Nivel_0_Seguridad_P5] -> HMI_ESTADO_16/1
  [TOP_Nivel_0_Seguridad_P5] -> LOG_n0_brakeHoistOpen/1
  [TOP_Nivel_0_Seguridad_P6] -> HMI_ESTADO_17/1
  [TOP_Nivel_0_Seguridad_P6] -> LOG_n0_emergencyBrakeHoistOpen/1
  [TOP_Nivel_0_Seguridad_P7] -> HMI_ESTADO_22/1
  [TOP_Nivel_0_Seguridad_P7] -> LOG_n0_emergency/1
  [TOP_Nivel_0_Seguridad_P8] -> HMI_ESTADO_29/1
  [TOP_Nivel_0_Seguridad_P9] -> HMI_ESTADO_31/1
  [TOP_PICK_PLACE_P1] -> Memory/1
  [TOP_PICK_PLACE_P2] -> Memory1/1
  [TOP_PICK_PLACE_P3] -> Memory2/1
  [TOP_PICK_PLACE_P4] -> MASS_loaded_gate/2, MASS_latch_pick/2(loaded)
  [TOP_SENSORES_P10] -> TERM_SENSOR_10/1
  [TOP_SENSORES_P8] -> TERM_SENSOR_08/1
  [TOP_SENSORES_P9] -> TERM_SENSOR_09/1
  [TOP_SUP_AUTO_TARGET_X_RAW_P1] -> TERM_HMI_SUP_AUTO_TARGET_X_RAW/1
  [TOP_SUP_CMD_AUTO_START_RAW_P1] -> TERM_HMI_SUP_CMD_AUTO_START_RAW/1
  [TOP_SUP_CMD_AUTO_START_RAW_STEP_P1] -> SUP_CMD_AUTO_START_RAW/1
  [TOP_SUP_CMD_RESET_RAW_P1] -> TERM_HMI_SUP_CMD_RESET_RAW/1
  [TOP_SUP_CMD_START_RAW_P1] -> TERM_HMI_SUP_CMD_START_RAW/1
  [TOP_SUP_CMD_START_RAW_STEP_P1] -> SUP_CMD_START_RAW/1
  [TOP_SUP_CMD_STOP_RAW_P1] -> TERM_HMI_SUP_CMD_STOP_RAW/1
  [TOP_SUP_CONFIG_VALID_RAW_P1] -> Interfaz de entradas del supervisor/7(IN_07_configValid)
  [TOP_SUP_CONTACT_BOOL_P1] -> Interfaz de entradas del supervisor/9(IN_09_contact4)
  [TOP_SUP_FB_BOOL_7_P1] -> Interfaz de entradas del supervisor/11(IN_11_normalLimitXMin)
  [TOP_SUP_FB_BOOL_8_P1] -> Interfaz de entradas del supervisor/12(IN_12_normalLimitXMax)
  [TOP_SUP_MODE_AUTO_REQ_RAW_P1] -> TERM_HMI_SUP_MODE_AUTO_REQ_RAW/1
  [TOP_SUP_NOT_OPEN_P1] -> SUP_TWISTLOCK_CMD/2
  [TOP_SUP_SCAN_PROFILE_REQ_RAW_P1] -> TERM_HMI_SUP_SCAN_PROFILE_REQ_RAW/1
  [TOP_SUP_SCAN_SPEED_RAW_P1] -> Interfaz de entradas del supervisor/33(IN_33_scanSpeed)
  [TOP_SUP_SWAY_SELECT_RAW_P1] -> Interfaz de entradas del supervisor/6(IN_06_swayControlSelect)
  [TOP_SUP_TLK_MEMORIA_P1] -> SUP_TLK_SET_OR/2
  [TOP_SUP_TLK_MEMORIA_P1] -> SUP_TWISTLOCK_FB_DELAY/1
  [TOP_SUP_TLK_SET_OR_P1] -> SUP_TWISTLOCK_CMD/1
  [TOP_SUP_TORQUE_HOIST_Z1_P1] -> Interfaz de entradas del supervisor/24(IN_24_torqueHoistRaw)
  [TOP_SUP_TORQUE_TROLLEY_Z1_P1] -> Interfaz de entradas del supervisor/23(IN_23_torqueTrolleyRaw)
  [TOP_SUP_TWISTLOCK_CMD_P1] -> SUP_TLK_DOUBLE/1
  [TOP_SUP_TWISTLOCK_CMD_P1] -> SUP_TLK_MEMORIA/1
  [TOP_SUP_TWISTLOCK_FB_DELAY_P1] -> Interfaz de entradas del supervisor/10(IN_10_twistlocksClosedFb)
  [TOP_Subsystem1_P1] -> HMI_SELECT_TWIST_BUTTON/1
  [TOP_Subsystem1_P2] -> HMI_SELECT_JOY_H/1
  [TOP_Subsystem1_P3] -> HMI_SELECT_JOY_T/1
  [TOP_Subsystem_P1] -> SUP_TORQUE_HOIST_Z1/1
  [TOP_Subsystem_P1] -> Zero-Order Hold9/1
  [TOP_Subsystem_P2] -> SUP_TORQUE_TROLLEY_Z1/1
  [TOP_Subsystem_P2] -> Zero-Order Hold10/1
  [TOP_Unit_Delay1_P1] -> SENSORES/8(TLK)
  [TOP_Unit_Delay_P1] -> Planta/6(TLK)
  [TOP_VISUALIZACION_2D_SISTEMA_GRUA_P10] -> HMI_MANDO_10/1
  [TOP_VISUALIZACION_2D_SISTEMA_GRUA_P11] -> HMI_MANDO_11/1
  [TOP_VISUALIZACION_2D_SISTEMA_GRUA_P12] -> HMI_MANDO_12/1
  [TOP_VISUALIZACION_2D_SISTEMA_GRUA_P13] -> HMI_RESERVA_13/1
  [TOP_VISUALIZACION_2D_SISTEMA_GRUA_P14] -> HMI_MANDO_14/1
  [TOP_VISUALIZACION_2D_SISTEMA_GRUA_P15] -> HMI_MANDO_15/1
  [TOP_VISUALIZACION_2D_SISTEMA_GRUA_P1] -> HMI_MANDO_01/1
  [TOP_VISUALIZACION_2D_SISTEMA_GRUA_P2] -> HMI_MANDO_02/1
  [TOP_VISUALIZACION_2D_SISTEMA_GRUA_P3] -> HMI_MANDO_03/1
  [TOP_VISUALIZACION_2D_SISTEMA_GRUA_P4] -> HMI_MANDO_04/1
  [TOP_VISUALIZACION_2D_SISTEMA_GRUA_P5] -> HMI_RESERVA_05/1
  [TOP_VISUALIZACION_2D_SISTEMA_GRUA_P6] -> HMI_MANDO_06/1
  [TOP_VISUALIZACION_2D_SISTEMA_GRUA_P7] -> HMI_RESERVA_07/1
  [TOP_VISUALIZACION_2D_SISTEMA_GRUA_P8] -> HMI_RESERVA_08/1
  [TOP_VISUALIZACION_2D_SISTEMA_GRUA_P9] -> HMI_MANDO_09/1
  [TOP_VIS_ZOH_01_P1] -> VISUALIZACION 2D SISTEMA GRUA/1
  [TOP_VIS_ZOH_02_P1] -> VISUALIZACION 2D SISTEMA GRUA/2
  [TOP_VIS_ZOH_03_P1] -> VISUALIZACION 2D SISTEMA GRUA/3
  [TOP_VIS_ZOH_04_P1] -> VISUALIZACION 2D SISTEMA GRUA/4
  [TOP_VIS_ZOH_05_P1] -> VISUALIZACION 2D SISTEMA GRUA/5
  [TOP_VIS_ZOH_06_P1] -> VISUALIZACION 2D SISTEMA GRUA/6
  [TOP_VIS_ZOH_07_P1] -> VISUALIZACION 2D SISTEMA GRUA/7
  [TOP_VIS_ZOH_08_P1] -> VISUALIZACION 2D SISTEMA GRUA/8
  [TOP_VIS_ZOH_09_P1] -> VISUALIZACION 2D SISTEMA GRUA/9
  [TOP_Zero_Order_Hold10_P1] -> Habilitacion par trolley/1
  [TOP_Zero_Order_Hold11_P1] -> Histeresis_contacto/1(F_cy)
  [TOP_Zero_Order_Hold12_P1] -> Histeresis_F_hw/1(F_hw)
  [TOP_Zero_Order_Hold9_P1] -> Habilitacion par izaje/1
  [TOP_slot_x_l_P1] -> MASS_slot_double/1
  [TOP_slot_x_l_P1] -> PICK / PLACE/2(k_slot)
  [TOP_slot_x_l_P2] -> PICK / PLACE/3(slot_ok)
  HMI_COLISION_NO_DISPONIBLE/1 -> [TOP_HMI_COLISION_NO_DISPONIBLE_P1]
  HMI_ESTADO_10/1 -> [TOP_HMI_ESTADO_10_P1]
  HMI_ESTADO_11/1 -> [TOP_HMI_ESTADO_11_P1]
  HMI_ESTADO_12/1 -> [TOP_HMI_ESTADO_12_P1]
  HMI_ESTADO_13/1 -> [TOP_HMI_ESTADO_13_P1]
  HMI_ESTADO_14/1 -> [TOP_HMI_ESTADO_14_P1]
  HMI_ESTADO_15/1 -> [TOP_HMI_ESTADO_15_P1]
  HMI_ESTADO_16/1 -> [TOP_HMI_ESTADO_16_P1]
  HMI_ESTADO_17/1 -> [TOP_HMI_ESTADO_17_P1]
  HMI_ESTADO_18/1 -> [TOP_HMI_ESTADO_18_P1]
  HMI_ESTADO_19/1 -> [TOP_HMI_ESTADO_19_P1]
  HMI_ESTADO_20/1 -> [TOP_HMI_ESTADO_20_P1]
  HMI_ESTADO_21/1 -> [TOP_HMI_ESTADO_21_P1]
  HMI_ESTADO_22/1 -> [TOP_HMI_ESTADO_22_P1]
  HMI_ESTADO_23/1 -> [TOP_HMI_ESTADO_23_P1]
  HMI_ESTADO_24/1 -> [TOP_HMI_ESTADO_24_P1]
  HMI_ESTADO_25/1 -> [TOP_HMI_ESTADO_25_P1]
  HMI_ESTADO_26/1 -> [TOP_HMI_ESTADO_26_P1]
  HMI_ESTADO_27/1 -> [TOP_HMI_ESTADO_27_P1]
  HMI_ESTADO_28/1 -> [TOP_HMI_ESTADO_28_P1]
  HMI_ESTADO_29/1 -> [TOP_HMI_ESTADO_29_P1]
  HMI_ESTADO_30/1 -> [TOP_HMI_ESTADO_30_P1]
  HMI_ESTADO_31/1 -> [TOP_HMI_ESTADO_31_P1]
  HMI_ESTADO_32/1 -> [TOP_HMI_ESTADO_32_P1]
  HMI_ESTADO_33/1 -> [TOP_HMI_ESTADO_33_P1]
  HMI_ESTADO_34/1 -> [TOP_HMI_ESTADO_34_P1]
  HMI_ESTADO_35/1 -> [TOP_HMI_ESTADO_35_P1]
  HMI_ESTADO_36/1 -> [TOP_HMI_ESTADO_36_P1]
  HMI_ESTADO_37/1 -> [TOP_HMI_ESTADO_37_P1]
  HMI_ESTADO_38/1 -> [TOP_HMI_ESTADO_38_P1]
  HMI_ESTADO_39/1 -> [TOP_HMI_ESTADO_39_P1]
  HMI_ESTADO_40/1 -> [TOP_HMI_ESTADO_40_P1]
  HMI_ESTADO_41/1 -> [TOP_HMI_ESTADO_41_P1]
  HMI_MANDO_01/1 -> [TOP_HMI_MANDO_01_P1]
  HMI_MANDO_02/1 -> [TOP_HMI_MANDO_02_P1]
  HMI_MANDO_03/1 -> [TOP_HMI_MANDO_03_P1]
  HMI_MANDO_04/1 -> [TOP_HMI_MANDO_04_P1]
  HMI_MANDO_06/1 -> [TOP_HMI_MANDO_06_P1]
  HMI_MANDO_09/1 -> [TOP_HMI_MANDO_09_P1]
  HMI_MANDO_10/1 -> [TOP_HMI_MANDO_10_P1]
  HMI_MANDO_11/1 -> [TOP_HMI_MANDO_11_P1]
  HMI_MANDO_12/1 -> [TOP_HMI_MANDO_12_P1]
  HMI_MANDO_14/1 -> [TOP_HMI_MANDO_14_P1]
  HMI_MANDO_15/1 -> [TOP_HMI_MANDO_15_P1]
  HMI_SELECT_JOY_H/1 -> [TOP_HMI_SELECT_JOY_H_P1]
  HMI_SELECT_JOY_T/1 -> [TOP_HMI_SELECT_JOY_T_P1]
  HMI_SELECT_TWIST_BUTTON/1 -> [TOP_HMI_SELECT_TWIST_BUTTON_P1]
  HMI_USE_JOYSTICK/1 -> [TOP_HMI_USE_JOYSTICK_P1]
  HMI_ZERO_INPUT/1 -> [TOP_HMI_ZERO_INPUT_P1]
  Habilitacion par izaje/1 -> [TOP_Habilitacion_par_izaje_P1]
  [SUP_ENABLE_HOIST] -> Habilitacion par izaje/2
  Habilitacion par trolley/1 -> [TOP_Habilitacion_par_trolley_P1]
  [SUP_ENABLE_TROLLEY] -> Habilitacion par trolley/2
  Histeresis_F_hw/1(tension) -> [TOP_Histeresis_F_hw_P1]  "tension"
  Histeresis_contacto/1(contacto) -> [TOP_Histeresis_contacto_P1]  "contacto"
  Interfaz de entradas del supervisor/1(OUT_01_cmdStart) -> [TOP_Interfaz_de_entradas_del_supervisor_P1]
  Interfaz de entradas del supervisor/2(OUT_02_cmdStop) -> [TOP_Interfaz_de_entradas_del_supervisor_P2]
  Interfaz de entradas del supervisor/3(OUT_03_modeAutoReq) -> [TOP_Interfaz_de_entradas_del_supervisor_P3]
  Interfaz de entradas del supervisor/4(OUT_04_cmdAutoStart) -> [TOP_Interfaz_de_entradas_del_supervisor_P4]
  Interfaz de entradas del supervisor/5(OUT_05_cmdReset) -> [TOP_Interfaz_de_entradas_del_supervisor_P5]
  Interfaz de entradas del supervisor/6(OUT_06_swayControlSelect) -> [TOP_Interfaz_de_entradas_del_supervisor_P6]
  Interfaz de entradas del supervisor/7(OUT_07_configValid) -> [TOP_Interfaz_de_entradas_del_supervisor_P7]
  Interfaz de entradas del supervisor/8(OUT_08_twistlockButton) -> [TOP_Interfaz_de_entradas_del_supervisor_P8]
  Interfaz de entradas del supervisor/9(OUT_09_contact4) -> [TOP_Interfaz_de_entradas_del_supervisor_P9]
  Interfaz de entradas del supervisor/10(OUT_10_twistlocksClosedFb) -> [TOP_Interfaz_de_entradas_del_supervisor_P10]
  Interfaz de entradas del supervisor/11(OUT_11_normalLimitXMin) -> [TOP_Interfaz_de_entradas_del_supervisor_P11]
  Interfaz de entradas del supervisor/12(OUT_12_normalLimitXMax) -> [TOP_Interfaz_de_entradas_del_supervisor_P12]
  Interfaz de entradas del supervisor/13(OUT_13_safetyPermitGlobal) -> [TOP_Interfaz_de_entradas_del_supervisor_P13]
  Interfaz de entradas del supervisor/14(OUT_14_safetyPermitTrolley) -> [TOP_Interfaz_de_entradas_del_supervisor_P14]
  Interfaz de entradas del supervisor/15(OUT_15_safetyPermitHoist) -> [TOP_Interfaz_de_entradas_del_supervisor_P15]
  Interfaz de entradas del supervisor/16(OUT_16_joyTrolley) -> [TOP_Interfaz_de_entradas_del_supervisor_P16]
  Interfaz de entradas del supervisor/17(OUT_17_joyHoist) -> [TOP_Interfaz_de_entradas_del_supervisor_P17]
  Interfaz de entradas del supervisor/18(OUT_18_xTrolley) -> [TOP_Interfaz_de_entradas_del_supervisor_P18]
  Interfaz de entradas del supervisor/19(OUT_19_omegaTrolley) -> [TOP_Interfaz_de_entradas_del_supervisor_P19]
  Interfaz de entradas del supervisor/20(OUT_20_yHoist) -> [TOP_Interfaz_de_entradas_del_supervisor_P20]
  Interfaz de entradas del supervisor/21(OUT_21_vHoist) -> [TOP_Interfaz_de_entradas_del_supervisor_P21]
  Interfaz de entradas del supervisor/22(OUT_22_ropeTension) -> [TOP_Interfaz_de_entradas_del_supervisor_P22]
  Interfaz de entradas del supervisor/23(OUT_23_torqueTrolleyRaw) -> [TOP_Interfaz_de_entradas_del_supervisor_P23]
  Interfaz de entradas del supervisor/24(OUT_24_torqueHoistRaw) -> [TOP_Interfaz_de_entradas_del_supervisor_P24]
  Interfaz de entradas del supervisor/25(OUT_25_autoTargetX) -> [TOP_Interfaz_de_entradas_del_supervisor_P25]
  Interfaz de entradas del supervisor/26(OUT_26_manualToAutoHeight) -> [TOP_Interfaz_de_entradas_del_supervisor_P26]
  Interfaz de entradas del supervisor/27(OUT_27_finalApproachDistance) -> [TOP_Interfaz_de_entradas_del_supervisor_P27]
  Interfaz de entradas del supervisor/28(OUT_28_spreaderSwayAngle) -> [TOP_Interfaz_de_entradas_del_supervisor_P28]
  Interfaz de entradas del supervisor/29(OUT_29_spreaderSwayRate) -> [TOP_Interfaz_de_entradas_del_supervisor_P29]
  Interfaz de entradas del supervisor/30(OUT_30_scanProfileReq) -> [TOP_Interfaz_de_entradas_del_supervisor_P30]
  Interfaz de entradas del supervisor/31(OUT_31_lidarX) -> [TOP_Interfaz_de_entradas_del_supervisor_P31]
  Interfaz de entradas del supervisor/32(OUT_32_lidarY) -> [TOP_Interfaz_de_entradas_del_supervisor_P32]
  Interfaz de entradas del supervisor/33(OUT_33_scanSpeed) -> [TOP_Interfaz_de_entradas_del_supervisor_P33]
  [x_t] -> LIDAR_OFFSET_X/1
  LIDAR_OFFSET_X/1 -> [TOP_LIDAR_OFFSET_X_P1]
  LIDAR_PROFILE_LOOKUP/1 -> [TOP_LIDAR_PROFILE_LOOKUP_P1]
  MASS_latch_pick/1(mass) -> [TOP_MASS_latch_pick_P1]
  MASS_loaded_gate/1 -> [TOP_MASS_loaded_gate_P1]
  MASS_profile_lookup/1 -> [TOP_MASS_profile_lookup_P1]
  MASS_slot_double/1 -> [TOP_MASS_slot_double_P1]
  Memory/1 -> [TOP_Memory_P1]  "evento_cambio"
  Memory1/1 -> [TOP_Memory1_P1]  "tipo_evento"
  Memory2/1 -> [TOP_Memory2_P1]  "slot_evento"
  N0_CMD_ESTOP/1 -> [TOP_N0_CMD_ESTOP_P1]
  N0_CMD_RESET/1 -> [TOP_N0_CMD_RESET_P1]
  [v_ly] -> Nivel 0 - Seguridad/7(vHoist)
  [x_td_est] -> Nivel 0 - Seguridad/4(xTrolley)
  [y_l] -> Nivel 0 - Seguridad/6(yHoist)
  N0_GATE_BRK_H/1 -> [TOP_N0_GATE_BRK_H_P1]
  N0_GATE_BRK_HE/1 -> [TOP_N0_GATE_BRK_HE_P1]
  [N0_BRK_HE] -> N0_GATE_BRK_HE/2
  [N0_BRK_H] -> N0_GATE_BRK_H/2
  N0_GATE_BRK_T/1 -> [TOP_N0_GATE_BRK_T_P1]
  [N0_BRK_T] -> N0_GATE_BRK_T/2
  N0_WATCHDOG_DELAY/1 -> [TOP_N0_WATCHDOG_DELAY_P1]
  N0_WATCHDOG_DOUBLE/1 -> [TOP_N0_WATCHDOG_DOUBLE_P1]
  Nivel 0 - Seguridad/1(permitGlobal) -> [N0_PERMIT_GLOBAL], [TOP_Nivel_0_Seguridad_P1]
  Nivel 0 - Seguridad/2(permitTrolley) -> [N0_PERMIT_TROLLEY], [TOP_Nivel_0_Seguridad_P2]
  Nivel 0 - Seguridad/3(permitHoist) -> [N0_PERMIT_HOIST], [TOP_Nivel_0_Seguridad_P3]
  Nivel 0 - Seguridad/4(brakeTrolleyOpen) -> [N0_BRK_T], [TOP_Nivel_0_Seguridad_P4]
  Nivel 0 - Seguridad/5(brakeHoistOpen) -> [N0_BRK_H], [TOP_Nivel_0_Seguridad_P5]
  Nivel 0 - Seguridad/6(emergencyBrakeHoistOpen) -> [N0_BRK_HE], [TOP_Nivel_0_Seguridad_P6]
  Nivel 0 - Seguridad/7(emergency) -> [TOP_Nivel_0_Seguridad_P7]
  Nivel 0 - Seguridad/8(hmiWatchdogFault) -> [TOP_Nivel_0_Seguridad_P8]
  Nivel 0 - Seguridad/9(hmiUltimate1) -> [TOP_Nivel_0_Seguridad_P9]
  Nivel 0 - Seguridad/10(hmiUltimate2) -> [TOP_Nivel_0_Seguridad_P10]
  Nivel 0 - Seguridad/11(hmiUltimate3) -> [TOP_Nivel_0_Seguridad_P11]
  Nivel 0 - Seguridad/12(hmiUltimate4) -> [TOP_Nivel_0_Seguridad_P12]
  PICK / PLACE/1(evento_cambio) -> [TOP_PICK_PLACE_P1]
  PICK / PLACE/2(tipo_evento) -> [TOP_PICK_PLACE_P2]
  PICK / PLACE/3(slot_evento) -> [TOP_PICK_PLACE_P3]
  PICK / PLACE/4(carga_tomada) -> [carga_tomada], [TOP_PICK_PLACE_P4]
  [Y_c] -> LIDAR_PROFILE_LOOKUP/2
  Planta/1(theta_tm) -> [theta_tm]
  Planta/2(theta_hm) -> [theta_hm]
  Planta/3(F_hw) -> [F_hw]
  Planta/4(theta_l) -> [theta_l]
  Planta/5(omega_l) -> [omega_l]
  Planta/6(omega_hd) -> [omega_hd]
  Planta/7(v_ly) -> [v_ly]
  Planta/8(x_l) -> [x_l]
  Planta/9(F_cy) -> [F_cy]
  Planta/10(x_t) -> [x_t]
  Planta/11(y_l) -> [y_l]
  SENSORES/1(theta_tm_sens) -> Interfaz MC/2(Encoder carro)
  SENSORES/2(theta_hm_sens) -> Interfaz MC/3(Encoder izaje)
  SENSORES/3(F_hw_sens) -> [F_hw_sens]  "F_hw_sens"
  SENSORES/4(omega_l_sens) -> [omega_l_sens]
  SENSORES/5(theta_l_sens) -> [theta_l_sens]
  SENSORES/6(x_tLSmin) -> [x_tLSmin]
  SENSORES/7(x_tLSmax) -> [x_tLSmax]
  SENSORES/8(x_tLSEmin) -> [TOP_SENSORES_P8]
  SENSORES/9(x_tLSEmax) -> [TOP_SENSORES_P9]
  SENSORES/10(Sobrevelocidad Izaje) -> [TOP_SENSORES_P10]
  [theta_l_sens] -> Interfaz de entradas del supervisor/28(IN_28_spreaderSwayAngle)
  [omega_l_sens] -> Interfaz de entradas del supervisor/29(IN_29_spreaderSwayRate)
  SUP_AUTO_TARGET_X_RAW/1 -> [TOP_SUP_AUTO_TARGET_X_RAW_P1]
  [SUP_BRAKE_H_OPEN] -> N0_GATE_BRK_H/1
  [SUP_BRAKE_HE_OPEN] -> N0_GATE_BRK_HE/1
  [SUP_BRAKE_T_OPEN] -> N0_GATE_BRK_T/1
  SUP_CMD_AUTO_START_RAW/1 -> [TOP_SUP_CMD_AUTO_START_RAW_P1]
  SUP_CMD_AUTO_START_RAW_STEP/1 -> [TOP_SUP_CMD_AUTO_START_RAW_STEP_P1]
  SUP_CMD_RESET_RAW/1 -> [TOP_SUP_CMD_RESET_RAW_P1]
  SUP_CMD_START_RAW/1 -> [TOP_SUP_CMD_START_RAW_P1]
  SUP_CMD_START_RAW_STEP/1 -> [TOP_SUP_CMD_START_RAW_STEP_P1]
  SUP_CMD_STOP_RAW/1 -> [TOP_SUP_CMD_STOP_RAW_P1]
  SUP_CONFIG_VALID_RAW/1 -> [TOP_SUP_CONFIG_VALID_RAW_P1]
  SUP_CONTACT_BOOL/1 -> [TOP_SUP_CONTACT_BOOL_P1]
  [x_td_est] -> Interfaz de entradas del supervisor/18(IN_18_xTrolley)
  [omega_td_est] -> Interfaz de entradas del supervisor/19(IN_19_omegaTrolley)
  [y_l] -> Interfaz de entradas del supervisor/20(IN_20_yHoist)
  [v_ly] -> Interfaz de entradas del supervisor/21(IN_21_vHoist)
  [F_hw_sens] -> Interfaz de entradas del supervisor/22(IN_22_ropeTension)
  [carga_tomada] -> TERM_SUP_FB_6/1
  [x_tLSmin] -> SUP_FB_BOOL_7/1
  [x_tLSmax] -> SUP_FB_BOOL_8/1
  SUP_FB_BOOL_7/1 -> [TOP_SUP_FB_BOOL_7_P1]
  SUP_FB_BOOL_8/1 -> [TOP_SUP_FB_BOOL_8_P1]
  SUP_MODE_AUTO_REQ_RAW/1 -> [TOP_SUP_MODE_AUTO_REQ_RAW_P1]
  SUP_NOT_OPEN/1 -> [TOP_SUP_NOT_OPEN_P1]
  [N0_PERMIT_GLOBAL] -> Interfaz de entradas del supervisor/13(IN_13_safetyPermitGlobal)
  [N0_PERMIT_HOIST] -> Interfaz de entradas del supervisor/15(IN_15_safetyPermitHoist)
  [N0_PERMIT_TROLLEY] -> Interfaz de entradas del supervisor/14(IN_14_safetyPermitTrolley)
  SUP_SCAN_PROFILE_REQ_RAW/1 -> [TOP_SUP_SCAN_PROFILE_REQ_RAW_P1]
  SUP_SCAN_SPEED_RAW/1 -> [TOP_SUP_SCAN_SPEED_RAW_P1]
  SUP_SWAY_SELECT_RAW/1 -> [TOP_SUP_SWAY_SELECT_RAW_P1]
  SUP_TLK_DOUBLE/1 -> [SUP_TLK]
  [SUP_TLK] -> [TLK]
  SUP_TLK_MEMORIA/1 -> [TOP_SUP_TLK_MEMORIA_P1]
  SUP_TLK_SET_OR/1 -> [TOP_SUP_TLK_SET_OR_P1]
  SUP_TORQUE_HOIST_Z1/1 -> [TOP_SUP_TORQUE_HOIST_Z1_P1]
  SUP_TORQUE_TROLLEY_Z1/1 -> [TOP_SUP_TORQUE_TROLLEY_Z1_P1]
  SUP_TWISTLOCK_CMD/1 -> [TOP_SUP_TWISTLOCK_CMD_P1]
  SUP_TWISTLOCK_FB_DELAY/1 -> [TOP_SUP_TWISTLOCK_FB_DELAY_P1]
  Motion Controller/1(T_hm*) -> [TOP_Subsystem_P1]
  Motion Controller/2(T_tmcontrolador) -> [TOP_Subsystem_P2]
  Subsystem1/1(boton) -> [TOP_Subsystem1_P1]
  Subsystem1/2(joy_vert) -> [TOP_Subsystem1_P2]
  Subsystem1/3(joy_hor) -> [TOP_Subsystem1_P3]
  Unit Delay/1 -> [TOP_Unit_Delay_P1]
  Unit Delay1/1 -> [TOP_Unit_Delay1_P1]
  [x_t] -> VIS ZOH 01/1
  [x_l] -> VIS ZOH 02/1
  [y_l] -> VIS ZOH 03/1
  [theta_l] -> VIS ZOH 04/1
  [SUP_TLK] -> VIS ZOH 05/1
  [Y_c] -> VIS ZOH 06/1
  [k_slot] -> VIS ZOH 07/1
  [yc_xl] -> VIS ZOH 08/1
  [carga_tomada] -> VIS ZOH 09/1
  VIS ZOH 01/1 -> [TOP_VIS_ZOH_01_P1]
  VIS ZOH 02/1 -> [TOP_VIS_ZOH_02_P1]
  VIS ZOH 03/1 -> [TOP_VIS_ZOH_03_P1]
  VIS ZOH 04/1 -> [TOP_VIS_ZOH_04_P1]
  VIS ZOH 05/1 -> [TOP_VIS_ZOH_05_P1]
  VIS ZOH 06/1 -> [TOP_VIS_ZOH_06_P1]
  VIS ZOH 07/1 -> [TOP_VIS_ZOH_07_P1]
  VIS ZOH 08/1 -> [TOP_VIS_ZOH_08_P1]
  VIS ZOH 09/1 -> [TOP_VIS_ZOH_09_P1]
  VISUALIZACION 2D SISTEMA GRUA/1 -> [TOP_VISUALIZACION_2D_SISTEMA_GRUA_P1]
  VISUALIZACION 2D SISTEMA GRUA/2 -> [TOP_VISUALIZACION_2D_SISTEMA_GRUA_P2]
  VISUALIZACION 2D SISTEMA GRUA/3 -> [TOP_VISUALIZACION_2D_SISTEMA_GRUA_P3]
  VISUALIZACION 2D SISTEMA GRUA/4 -> [TOP_VISUALIZACION_2D_SISTEMA_GRUA_P4]
  VISUALIZACION 2D SISTEMA GRUA/5 -> [TOP_VISUALIZACION_2D_SISTEMA_GRUA_P5]
  VISUALIZACION 2D SISTEMA GRUA/6 -> [TOP_VISUALIZACION_2D_SISTEMA_GRUA_P6]
  VISUALIZACION 2D SISTEMA GRUA/7 -> [TOP_VISUALIZACION_2D_SISTEMA_GRUA_P7]
  VISUALIZACION 2D SISTEMA GRUA/8 -> [TOP_VISUALIZACION_2D_SISTEMA_GRUA_P8]
  VISUALIZACION 2D SISTEMA GRUA/9 -> [TOP_VISUALIZACION_2D_SISTEMA_GRUA_P9]
  VISUALIZACION 2D SISTEMA GRUA/10 -> [TOP_VISUALIZACION_2D_SISTEMA_GRUA_P10]
  VISUALIZACION 2D SISTEMA GRUA/11 -> [TOP_VISUALIZACION_2D_SISTEMA_GRUA_P11]
  VISUALIZACION 2D SISTEMA GRUA/12 -> [TOP_VISUALIZACION_2D_SISTEMA_GRUA_P12]
  VISUALIZACION 2D SISTEMA GRUA/13 -> [TOP_VISUALIZACION_2D_SISTEMA_GRUA_P13]
  VISUALIZACION 2D SISTEMA GRUA/14 -> [TOP_VISUALIZACION_2D_SISTEMA_GRUA_P14]
  VISUALIZACION 2D SISTEMA GRUA/15 -> [TOP_VISUALIZACION_2D_SISTEMA_GRUA_P15]
  Zero-Order Hold/1 -> [TOP_Zero_Order_Hold_P1]
  Zero-Order Hold10/1 -> [TOP_Zero_Order_Hold10_P1]
  Zero-Order Hold11/1 -> [TOP_Zero_Order_Hold11_P1]
  Zero-Order Hold12/1 -> [TOP_Zero_Order_Hold12_P1]
  Zero-Order Hold5/1 -> Interfaz MC/4(Angulo balanceo)
  Zero-Order Hold6/1 -> [TOP_Zero_Order_Hold6_P1]
  Zero-Order Hold7/1 -> [TOP_Zero_Order_Hold7_P1]
  Zero-Order Hold8/1 -> [TOP_Zero_Order_Hold8_P1]
  Zero-Order Hold9/1 -> [TOP_Zero_Order_Hold9_P1]
  slot_x_l/1(k_slot) -> [k_slot], [TOP_slot_x_l_P1]
  slot_x_l/2(slot_ok) -> [TOP_slot_x_l_P2]
  Motion Controller/3(SW aplicada comun) -> SW ultima muestra N1/1
  Planta/12(Delta torque limite carro) -> Memoria recorte torque AW/1
  [TOP_Zero_Order_Hold_P1] -> Interfaz MC/1(Tension cable)
  [TOP_Zero_Order_Hold6_P1] -> Interfaz MC/5(xRef)
  [TOP_Zero_Order_Hold7_P1] -> Interfaz MC/6(vRef)
  [TOP_Zero_Order_Hold8_P1] -> Interfaz MC/7(aRef)
  Memoria recorte torque AW/1 -> Interfaz MC/13(Recorte torque demorado)
  Interfaz MC/1(Sensors) -> Motion Controller/1(Sensors)
  Interfaz MC/2(References) -> Motion Controller/2(References)
  Interfaz MC/3(Commands) -> Motion Controller/3(Commands)
  Interfaz MC/4(Drive Feedback) -> Motion Controller/4(Drive Feedback)
  Motion Controller/4(Estados carro) -> Estados MC carro/1
  Motion Controller/5(Estados izaje) -> Estados MC izaje/1
  Estados MC carro/1 -> Monitor estado carro 1/1, [x_td_est]  "<x>"
  Estados MC izaje/1 -> Monitor estado izaje 1/1  "<length>"
  Estados MC carro/2 -> Monitor estado carro 2/1, [omega_td_est]  "<omegaDrum>"
  Estados MC izaje/2 -> Monitor estado izaje 2/1  "<lengthRate>"
  Estados MC carro/3 -> Monitor estado carro 3/1, [TOP_N0_OMEGA_A_VT_P1]  "<velocity>"
  Estados MC izaje/3 -> Monitor estado izaje 3/1  "<omegaDrum>"
  Estados MC carro/4 -> Monitor estado carro 4/1  "<observerAngle>"
  Estados MC izaje/4 -> Monitor estado izaje 4/1  "<observerAngle>"
  Motion Controller/6(Diagnosticos carro) -> Monitor bus diagnosticos 6/1
  Motion Controller/7(Diagnosticos izaje) -> Monitor bus diagnosticos 7/1
  [TOP_Interfaz_de_entradas_del_supervisor_P1] -> Automata Supervisor/1(cmdStart)
  [TOP_Interfaz_de_entradas_del_supervisor_P2] -> Automata Supervisor/2(cmdStop)
  [TOP_Interfaz_de_entradas_del_supervisor_P3] -> Automata Supervisor/3(modeAutoReq)
  [TOP_Interfaz_de_entradas_del_supervisor_P4] -> Automata Supervisor/4(cmdAutoStart)
  [TOP_Interfaz_de_entradas_del_supervisor_P5] -> Automata Supervisor/5(cmdReset)
  [TOP_Interfaz_de_entradas_del_supervisor_P6] -> Automata Supervisor/6(swayControlSelect)
  [TOP_Interfaz_de_entradas_del_supervisor_P7] -> Automata Supervisor/7(configValid)
  [TOP_Interfaz_de_entradas_del_supervisor_P8] -> Automata Supervisor/8(twistlockButton)
  [TOP_Interfaz_de_entradas_del_supervisor_P9] -> Automata Supervisor/9(contact4)
  [TOP_Interfaz_de_entradas_del_supervisor_P10] -> Automata Supervisor/10(twistlocksClosedFb)
  [TOP_Interfaz_de_entradas_del_supervisor_P11] -> Automata Supervisor/11(normalLimitXMin)
  [TOP_Interfaz_de_entradas_del_supervisor_P12] -> Automata Supervisor/12(normalLimitXMax)
  [TOP_Interfaz_de_entradas_del_supervisor_P13] -> Automata Supervisor/13(safetyPermitGlobal)
  [TOP_Interfaz_de_entradas_del_supervisor_P14] -> Automata Supervisor/14(safetyPermitTrolley)
  [TOP_Interfaz_de_entradas_del_supervisor_P15] -> Automata Supervisor/15(safetyPermitHoist)
  [TOP_Interfaz_de_entradas_del_supervisor_P16] -> Automata Supervisor/16(joyTrolley)
  [TOP_Interfaz_de_entradas_del_supervisor_P17] -> Automata Supervisor/17(joyHoist)
  [TOP_Interfaz_de_entradas_del_supervisor_P18] -> Automata Supervisor/18(xTrolley)
  [TOP_Interfaz_de_entradas_del_supervisor_P19] -> Automata Supervisor/19(omegaTrolley)
  [TOP_Interfaz_de_entradas_del_supervisor_P20] -> Automata Supervisor/20(yHoist)
  [TOP_Interfaz_de_entradas_del_supervisor_P21] -> Automata Supervisor/21(vHoist)
  [TOP_Interfaz_de_entradas_del_supervisor_P22] -> Automata Supervisor/22(ropeTension)
  [TOP_Interfaz_de_entradas_del_supervisor_P23] -> Automata Supervisor/23(torqueTrolleyRaw)
  [TOP_Interfaz_de_entradas_del_supervisor_P24] -> Automata Supervisor/24(torqueHoistRaw)
  [TOP_Interfaz_de_entradas_del_supervisor_P25] -> Automata Supervisor/25(autoTargetX)
  [TOP_Interfaz_de_entradas_del_supervisor_P26] -> Automata Supervisor/26(manualToAutoHeight)
  [TOP_Interfaz_de_entradas_del_supervisor_P27] -> Automata Supervisor/27(finalApproachDistance)
  [TOP_Interfaz_de_entradas_del_supervisor_P28] -> Automata Supervisor/28(spreaderSwayAngle)
  [TOP_Interfaz_de_entradas_del_supervisor_P29] -> Automata Supervisor/29(spreaderSwayRate)
  [TOP_Interfaz_de_entradas_del_supervisor_P30] -> Automata Supervisor/30(hmiScanRequestRaw)
  [TOP_Interfaz_de_entradas_del_supervisor_P31] -> Automata Supervisor/31(lidarX)
  [TOP_Interfaz_de_entradas_del_supervisor_P32] -> Automata Supervisor/32(lidarY)
  [TOP_Interfaz_de_entradas_del_supervisor_P33] -> Automata Supervisor/33(scanSpeed)
  Automata Supervisor/1(enableTrolleyReg) -> [SUP_ENABLE_TROLLEY]  "x_gen"
  Automata Supervisor/2(enableHoistReg) -> [SUP_ENABLE_HOIST]
  Automata Supervisor/3(brakeTrolleyOpenCmd) -> [SUP_BRAKE_T_OPEN], Interfaz MC/10(Freno carro abierto)
  Automata Supervisor/4(brakeHoistOpenCmd) -> [SUP_BRAKE_H_OPEN]
  Automata Supervisor/5(emergencyBrakeHoistOpenCmd) -> [SUP_BRAKE_HE_OPEN]  "dx_gen"
  Automata Supervisor/6(twistlockCloseCmd) -> [TOP_Automata_Supervisor_P6]
  Automata Supervisor/7(twistlockOpenCmd) -> [TOP_Automata_Supervisor_P7]
  Automata Supervisor/8(swayControlEnable) -> Interfaz MC/11(E antisway), [TOP_Automata_Supervisor_P8]
  Automata Supervisor/9(loadedState) -> [TOP_Automata_Supervisor_P9]
  Automata Supervisor/10(overloadDetected) -> [TOP_Automata_Supervisor_P10]
  Automata Supervisor/11(watchdogToggle) -> [TOP_Automata_Supervisor_P11]
  Automata Supervisor/12(xRef) -> [x_tgen]  "yl_gen"
  Automata Supervisor/13(vxRef) -> [v_tgen]
  Automata Supervisor/14(axRef) -> [a_tgen]
  Automata Supervisor/15(yRef) -> [TOP_Automata_Supervisor_P15]
  Automata Supervisor/16(vyRef) -> [TOP_Automata_Supervisor_P16], Interfaz MC/8(Velocidad izaje ref)
  Automata Supervisor/17(ayRef) -> [TOP_Automata_Supervisor_P17], Interfaz MC/9(Aceleracion izaje ref)
  Automata Supervisor/18(modeCode) -> [TOP_Automata_Supervisor_P18]
  Automata Supervisor/19(alarmCode) -> [TOP_Automata_Supervisor_P19]
  Automata Supervisor/20(faultCode) -> [TOP_Automata_Supervisor_P20]
  Automata Supervisor/21(aTrolley) -> [TOP_Automata_Supervisor_P21]
  Automata Supervisor/22(aHoist) -> [TOP_Automata_Supervisor_P22]
  Automata Supervisor/23(trackingFault) -> [TOP_Automata_Supervisor_P23]
  Automata Supervisor/24(torqueProvenTrolley) -> [TOP_Automata_Supervisor_P24]
  Automata Supervisor/25(torqueProvenHoist) -> [TOP_Automata_Supervisor_P25]
  Automata Supervisor/26(profileScanComplete) -> [TOP_Automata_Supervisor_P26]
  Automata Supervisor/27(profileValid) -> [TOP_Automata_Supervisor_P27]
  Automata Supervisor/28(scanActive) -> [TOP_Automata_Supervisor_P28]
  Automata Supervisor/29(scannedObstacleProfile) -> [TOP_Automata_Supervisor_P29]
  Automata Supervisor/30(profileMaxY) -> [TOP_Automata_Supervisor_P30]
  Automata Supervisor/31(automaticTargetY) -> [TOP_Automata_Supervisor_P31]
  Automata Supervisor/32(clearanceLineY) -> [TOP_Automata_Supervisor_P32]
  Automata Supervisor/33(estimatedContainerMass) -> [TOP_Automata_Supervisor_P33]
  Automata Supervisor/34(massEstimateValid) -> [TOP_Automata_Supervisor_P34]
  Automata Supervisor/35(normalLimitYMin) -> [TOP_Automata_Supervisor_P35]
  Automata Supervisor/36(normalLimitYMax) -> [TOP_Automata_Supervisor_P36]
  Automata Supervisor/37(manualTrolleyRef) -> [TOP_Automata_Supervisor_P37]
  Automata Supervisor/38(manualHoistRef) -> [TOP_Automata_Supervisor_P38]
  Automata Supervisor/39(safetyEnvelopeProfile) -> VISUALIZACION 2D SISTEMA GRUA/42, Registrar_envolvente_seguridad/1
  SW ultima muestra N1/1 -> Transferencia antisway no transmitida/1
  Transferencia no implementada PLC anterior/1 -> Interfaz MC/12(Transferencia SW)
